simulink model "first"  (R2016a)
settings: Solver=VariableStepAuto  StartTime=0.0  StopTime=10.0  RelTol=1e-3
settings Model: Creator=kypis  LastModifiedBy=kypis

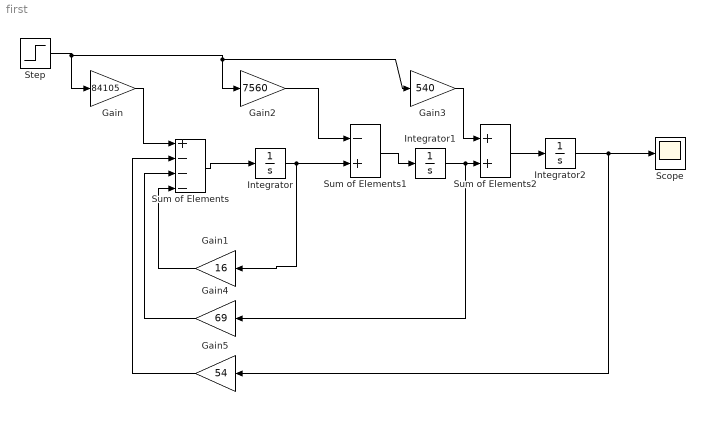
== system first ==
  Gain : Gain  Gain=84105
  Gain1 : Gain  Gain=16
  Gain2 : Gain  Gain=7560
  Gain3 : Gain  Gain=540
  Gain4 : Gain  Gain=69
  Gain5 : Gain  Gain=54
  Integrator : Integrator
  Integrator1 : Integrator
  Integrator2 : Integrator
  Scope : Scope
  Step : Step  Time=0  SampleTime=0
  Sum of Elements : Sum  Inputs=+---
  Sum of Elements1 : Sum  Inputs=-+
  Sum of Elements2 : Sum
  wires:
  Step/1 -> Gain3/1, Gain2/1, Gain/1
  Gain/1 -> Sum of Elements/1
  Sum of Elements/1 -> Integrator/1
  Integrator/1 -> Gain1/1, Sum of Elements1/2
  Gain1/1 -> Sum of Elements/4
  Integrator2/1 -> Gain5/1, Scope/1
  Sum of Elements1/1 -> Integrator1/1
  Gain2/1 -> Sum of Elements1/1
  Sum of Elements2/1 -> Integrator2/1
  Gain3/1 -> Sum of Elements2/1
  Integrator1/1 -> Gain4/1, Sum of Elements2/2
  Gain4/1 -> Sum of Elements/3
  Gain5/1 -> Sum of Elements/2
